simulink model "p2_sim"  (R2025b)
settings: Solver=VariableStepAuto  StartTime=0.0  StopTime=inf  MaxStep=1/20e3  RelTol=1e-3
values from neighbouring files (symbols this model uses):
  AZ1 = 0.2    [p2_ini.m]
  omegaZ1 = omega0    (= 47.0611)    [p2_ini.m]
libraries: cstblocks x3
settings Model: Creator=pmic  LastModifiedBy=andre
settings SolverCC: AlgebraicLoopSolver=TrustRegion
settings DebuggingCC: UnconnectedInputMsg=warning  UnconnectedOutputMsg=warning  UnconnectedLineMsg=warning
settings ModelReferenceCC: EnableRefExpFcnMdlSchedulingChecks=on
settings RTWCC: GPUComputeCapability=3.5  DLArmComputeVersion=19.05

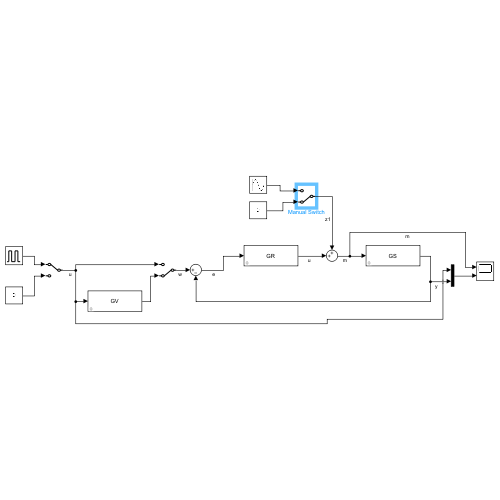
[thumbnail: Simulink's stored preview of the top-level diagram]
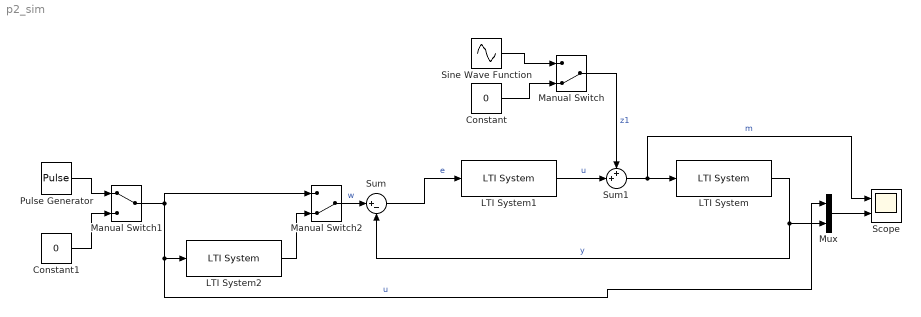
== system p2_sim ==
  Constant : Constant  Value=0
  Constant1 : Constant  Value=0
  LTI System : cstblocks/LTI System  sys=GS  IC=[]  PadeOrder=0
  LTI System1 : cstblocks/LTI System  sys=GR  IC=[]  PadeOrder=0
  LTI System2 : cstblocks/LTI System  sys=GV  IC=[]  PadeOrder=0
  Manual Switch : ManualSwitch  CurrentSetting=0
  Manual Switch1 : ManualSwitch
  Manual Switch2 : ManualSwitch  CurrentSetting=0
  Mux : Mux  Inputs=2
  Pulse Generator : DiscretePulseGenerator  PulseType=Time based  Period=0.5  PulseWidth=50  PhaseDelay=2
  Scope : Scope  NumInputPorts=2
      settings: ActiveDisplayYMinimum=-7.6130912947111842  ActiveDisplayYMaximum=4.4056921642568465
  Sine Wave Function : Sin  Amplitude=AZ1  Frequency=omegaZ1  SampleTime=0
  Sum : Sum  Inputs=|+-
  Sum1 : Sum  Inputs=++|
  wires:
  LTI System/1 -> Sum/2, Mux/2  "y"
  Constant/1 -> Manual Switch/2
  Sine Wave Function/1 -> Manual Switch/1
  Manual Switch1/1 -> LTI System2/1, Mux/1, Manual Switch2/1  "u"
  LTI System2/1 -> Manual Switch2/2
  Constant1/1 -> Manual Switch1/2
  Pulse Generator/1 -> Manual Switch1/1
  Mux/1 -> Scope/2
  LTI System1/1 -> Sum1/2  "u"
  Sum1/1 -> LTI System/1, Scope/1  "m"
  Sum/1 -> LTI System1/1  "e"
  Manual Switch/1 -> Sum1/1  "z1"
  Manual Switch2/1 -> Sum/1  "w"
